simulink model "rep3_transc_analysis_pulse"  (R2015a)
settings: Solver=ode4  StartTime=0.0  StopTime=1000  FixedStep=0.1  RelTol=1e-3
values from neighbouring files (symbols this model uses):
  c1 = 1.6    [rep3_transc_analysis_init.m]
  c2 = 0.12    [rep3_transc_analysis_init.m]
  K_D = 1    [rep3_transc_analysis_init.m]
  n0 = 0.5    [rep3_transc_analysis_init.m]
  n1 = 2    [rep3_transc_analysis_init.m]
  n2 = 4    [rep3_transc_analysis_init.m]
libraries: fuzblock x3
settings Model: Creator=jureb  LastModifiedBy=jure

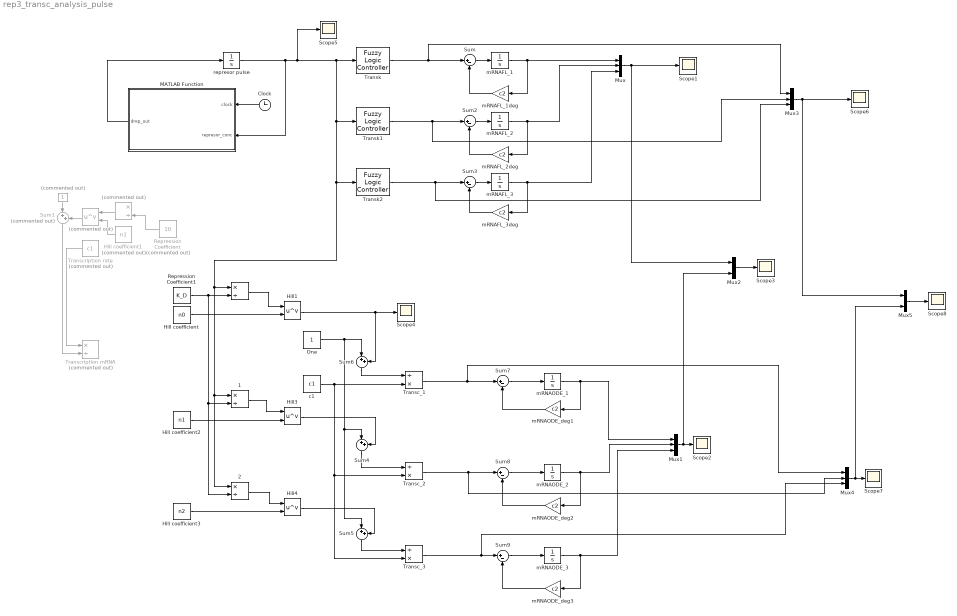
== system rep3_transc_analysis_pulse ==
  " " : Math  Commented=on  Operator=pow  SaturateOnIntegerOverflow=on
  " " : Product  Commented=on  Inputs=*/
  " " : Product  Inputs=*/
  " 1" : Product  Inputs=*/
  " 2" : Product  Inputs=*/
  "          " : Constant  Commented=on
  Clock : Clock
  Hill coefficient : Constant  Value=n0
  Hill coefficient1 : Constant  Commented=on  Value=n1
  Hill coefficient2 : Constant  Value=n1
  Hill coefficient3 : Constant  Value=n2
  Hill1 : Math  Operator=pow  SaturateOnIntegerOverflow=on
  Hill3 : Math  Operator=pow  SaturateOnIntegerOverflow=on
  Hill4 : Math  Operator=pow  SaturateOnIntegerOverflow=on
  MATLAB Function : MATLAB Function  TreatAsAtomicUnit=on
  Mux{,1,3..4} (4 alike) : Mux  Inputs=3
  Mux2 : Mux  Inputs=2
  Mux5 : Mux  Inputs=2
  One : Constant
  Repression Coefficient : Constant  Commented=on  Value=10
  Repression Coefficient1 : Constant  Value=K_D
  Scope{1..8} (8 alike) : Scope
      Scope1 settings: TimeRange=100  YMin=6.24957  YMax=6.25  SaveName=mRNA_FL_pulse
      Scope2 settings: TimeRange=100  YMin=0  YMax=1.5  SaveName=mRNA_ODE_pulse
      Scope3 settings: TimeRange=1000  YMin=0  YMax=18  SaveName=mRNAChange2
      Scope4 settings: TimeRange=100  YMin=0  YMax=1.5  SaveName=mRNAChange3
      Scope5 settings: TimeRange=100  YMin=0  YMax=1.5  SaveName=mRNAChange4
      Scope6 settings: TimeRange=100  YMin=6.24957  YMax=6.25  SaveName=mRNAc_FL_pulse
      Scope7 settings: TimeRange=100  YMin=0  YMax=1.5  SaveName=mRNAc_ODE_pulse
      Scope8 settings: TimeRange=1000  YMin=0  YMax=18  SaveName=mRNAChange
  Sum{,2..3,7..9} (6 alike) : Sum  Inputs=|+-
  Sum1 : Sum  Commented=on  Inputs=|++
  Sum4 : Sum  Inputs=|++
  Sum5 : Sum  Inputs=|++
  Sum6 : Sum  Inputs=|++
  Transc_1 : Product  Inputs=/*
  Transc_2 : Product  Inputs=/*
  Transc_3 : Product  Inputs=/*
  Transcription mRNA : Product  Commented=on  Inputs=*/
  Transcription rate : Constant  Commented=on  Value=c1
  Transk : fuzblock/Fuzzy Logic  Controller  fis=Transk0
  Transk1 : fuzblock/Fuzzy Logic  Controller  fis=Transk1
  Transk2 : fuzblock/Fuzzy Logic  Controller  fis=Transk2
  c1 : Constant  Value=c1
  mRNAFL_1 : Integrator  LimitOutput=on  LowerSaturationLimit=0
  mRNAFL_1deg : Gain  Gain=c2
  mRNAFL_2 : Integrator  LimitOutput=on  LowerSaturationLimit=0
  mRNAFL_2deg : Gain  Gain=c2
  mRNAFL_3 : Integrator  LimitOutput=on  LowerSaturationLimit=0
  mRNAFL_3deg : Gain  Gain=c2
  mRNAODE_1 : Integrator  LimitOutput=on  LowerSaturationLimit=0
  mRNAODE_2 : Integrator  LimitOutput=on  LowerSaturationLimit=0
  mRNAODE_3 : Integrator  LimitOutput=on  LowerSaturationLimit=0
  mRNAODE_deg1 : Gain  Gain=c2
  mRNAODE_deg2 : Gain  Gain=c2
  mRNAODE_deg3 : Gain  Gain=c2
  represor pulse : Integrator  InitialCondition=400  LimitOutput=on  UpperSaturationLimit=400  LowerSaturationLimit=0
  wires:
  Sum/1 -> mRNAFL_1/1
  mRNAFL_1/1 -> Mux/1, mRNAFL_1deg/1
  mRNAFL_1deg/1 -> Sum/2
  Mux/1 -> Mux2/1, Scope1/1
  One/1 -> Sum4/1, Sum5/1, Sum6/1
  Hill1/1 -> Scope4/1, Sum6/2
  Sum6/1 -> Transc_1/1
  c1/1 -> Transc_3/2, Transc_2/2, Transc_1/2
  Sum4/1 -> Transc_2/1
  Hill3/1 -> Sum4/2
  Hill coefficient3/1 -> Hill4/2
  Hill4/1 -> Sum5/2
  Sum5/1 -> Transc_3/1
  Mux1/1 -> Mux2/2, Scope2/1
  Mux2/1 -> Scope3/1
  Hill coefficient/1 -> Hill1/2
  Hill coefficient2/1 -> Hill3/2
  Sum1/1 -> Transcription mRNA/2
  "          "/1 -> Sum1/1
  Transcription rate/1 -> Transcription mRNA/1
  " "/1 -> Sum1/2
  Hill coefficient1/1 -> " "/2
  " "/1 -> " "/1
  Repression Coefficient/1 -> " "/2
  Sum2/1 -> mRNAFL_2/1
  mRNAFL_2/1 -> Mux/2, mRNAFL_2deg/1
  mRNAFL_2deg/1 -> Sum2/2
  Sum3/1 -> mRNAFL_3/1
  mRNAFL_3/1 -> Mux/3, mRNAFL_3deg/1
  mRNAFL_3deg/1 -> Sum3/2
  Sum7/1 -> mRNAODE_1/1
  mRNAODE_1/1 -> Mux1/1, mRNAODE_deg1/1
  mRNAODE_deg1/1 -> Sum7/2
  Sum8/1 -> mRNAODE_2/1
  mRNAODE_2/1 -> Mux1/2, mRNAODE_deg2/1
  mRNAODE_deg2/1 -> Sum8/2
  Sum9/1 -> mRNAODE_3/1
  mRNAODE_3/1 -> mRNAODE_deg3/1, Mux1/3
  mRNAODE_deg3/1 -> Sum9/2
  represor pulse/1 -> MATLAB Function/2(represor_conc), Transk/1, Transk1/1, " 2"/1, " 1"/1, " "/1, Transk2/1, Scope5/1
  MATLAB Function/1(drep_out) -> represor pulse/1
  Clock/1 -> MATLAB Function/1(clock)
  Repression Coefficient1/1 -> " 2"/2, " 1"/2, " "/2
  " "/1 -> Hill1/1
  " 2"/1 -> Hill4/1
  " 1"/1 -> Hill3/1
  Transk/1 -> Mux3/1, Sum/1
  Mux3/1 -> Mux5/1, Scope6/1
  Mux4/1 -> Mux5/2, Scope7/1
  Mux5/1 -> Scope8/1
  Transk1/1 -> Mux3/2, Sum2/1
  Transk2/1 -> Mux3/3, Sum3/1
  Transc_1/1 -> Mux4/1, Sum7/1
  Transc_2/1 -> Mux4/2, Sum8/1
  Transc_3/1 -> Mux4/3, Sum9/1

== matlab function rep3_transc_analysis_pulse/MATLAB Function ==
  data: clock input; drep_out output; represor_conc input
function drep_out  = degradation_transc_analysis(clock,represor_conc)

drep_out = 0;

if (clock < 400)
    drep_out = 0;    
elseif (clock >=400 && clock <=700)
    drep_out = -0.06*represor_conc;
else
    drep_out = 2.6*9-0.06*represor_conc;
end;
